simulink model "reconfig_dev_2021a"  (R2021a)
settings: Solver=VariableStepAuto  StartTime=0.0  StopTime=tsim  RelTol=1e-3
InitFcn:
  | main
values from neighbouring files (symbols this model uses):
  drone_params = get_parameters(1)    [main.m]
  dt = 0.005    [main.m]
  g = 9.81    [main.m]
  gust_duration = 5    [main.m]
  gust_force = [0;0;0]    [main.m]
  gust_start = 8    [main.m]
  omega0 = [[0,0,0]',[0,0,0]',[0,0,0]']    [main.m]
  p0 = [[0,0,2]',[0,0,2]',[0,0,2]']    [main.m]
  q0 = [[1,0,0,0]',[1,0,0,0]',[1,0,0,0]']    [main.m]
  tsim = 10    [main.m]
  v0 = [[0,0,0]',[0,0,0]',[0,0,0]']    [main.m]
libraries: vrlib x1
settings Model: Creator=gbattaglia2021  LastModifiedBy=Giacomo Battaglia

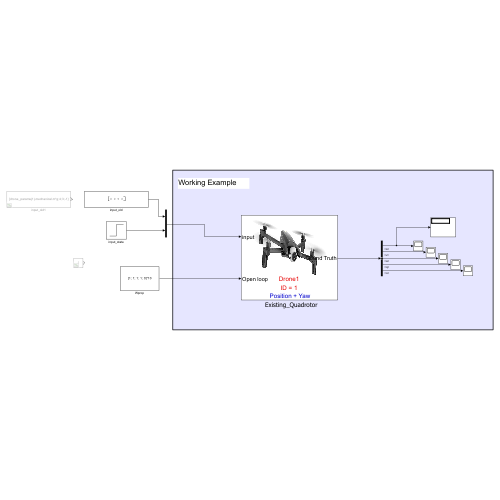
[thumbnail: Simulink's stored preview of the top-level diagram]
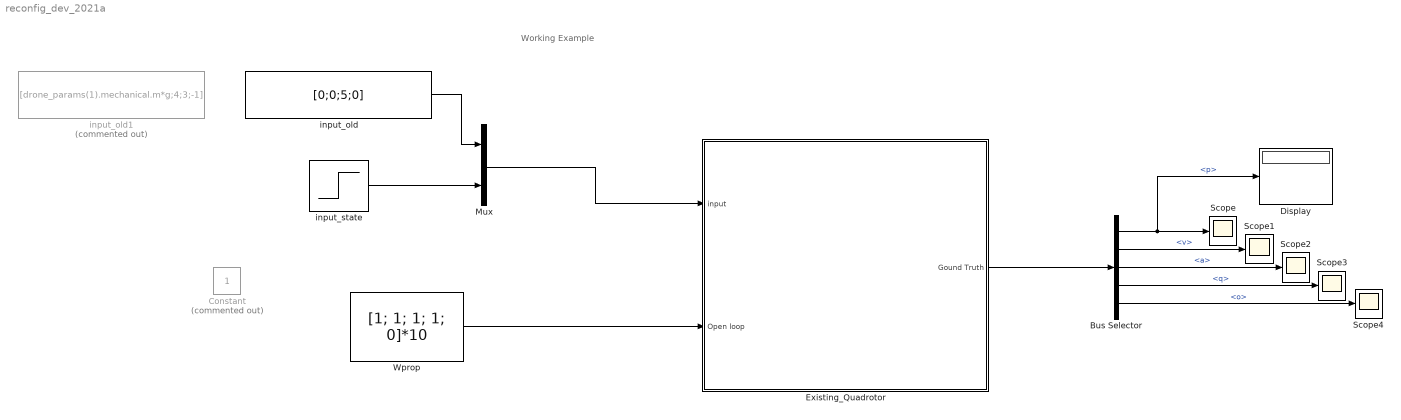
== system reconfig_dev_2021a ==
  note: Working Example
  "  Existing_Quadrotor" : Subsystem  mask{control_type_param=1: Position + Yaw, DroneID=1, DroneName=Drone1, idx_offset=0}
      mask prompts: control_type_param "Controller type"; DroneName "Drone Name"; idx_offset "Index Offset"
      mask TypeOptions control_type_param: 1: Position + Yaw | 2: Body Velocity + Yawrate | 3: Body Acceleration + Yawrate | 4: Thrust + Attitude | 5: Thrust + Body Rate | 6: Body Wrench
      mask TypeOptions DroneID: 1 | 2 | 3 | 4 | 5 | 6 | 7 | 8 | 9
      mask Callback DroneID:
      | ID = get_param(gcb,'DroneID');
      | offset = get_param(gcb,'idx_offset');
      | if ischar(ID)
      |   ID = str2num(ID);
      | end
      | if ischar(offset)
      |   offset = str2num(offset);
      | end
      | nameID = ID + offset;
      | set_param(gcb,'DroneName',["Drone"+num2str(nameID)]);
      mask Callback DroneName: set_param([gcb,'/To Workspace'],'VariableName',[get_param(gcb,'DroneName')]);
      mask Callback idx_offset:
      | ID = get_param(gcb,'DroneID');
      | offset = get_param(gcb,'idx_offset');
      | if ischar(ID)
      |   ID = str2num(ID);
      | end
      | if ischar(offset)
      |   offset = str2num(offset);
      | end
      | nameID = ID + offset;
      | set_param(gcb,'DroneName',["Drone"+num2str(nameID)]);
      mask DialogControl Control4 Prompt: click to choose controller
      mask Display:
      | image('format/drone_image.png'); % Use "Edit Image" on toolstrip to change.
      | Name = get_param(gcb,'DroneName');
      | ID = get_param(gcb,'DroneID');
      | C_mode = get_param(gcb,'control_type_param');
      | C_mode(1:2) = [];
      | color('red')
      | ID = "ID = "+ID;
      | color('red')
      | text(0.5, 0.25, Name, 'horizontalAlignment', 'center')
      | color('red')
      | text(0.5, 0.15, ID, 'horizontalAlignment', 'center')
      | color('blue');
      | text(0.5, 0.05, C_mode, 'horizontalAlignment', 'center')
  Bus Selector : BusSelector  OutputSignals=p,v,a,q,o
  Constant : Constant  Commented=on
  Display : Display
  Mux : Mux  Inputs=2
  Scope{,1..4} (5 alike) : Scope
  Wprop : Constant  Value=[1; 1; 1; 1; 0]*10
  input_old : Constant  Value=[0;0;5;0]
  input_old1 : Constant  Commented=on  Value=[drone_params(1).mechanical.m*g;4;3;-1]
  input_state : Step  Time=tsim/2  Before=drone_params(1).control.state  After=drone_params(1).control.state_enum.folded2  SampleTime=0
  wires:
  Bus Selector/1 -> Display/1, Scope/1  "<p>"
  Bus Selector/4 -> Scope3/1  "<q>"
  Bus Selector/5 -> Scope4/1  "<o>"
  Bus Selector/2 -> Scope1/1  "<v>"
  "  Existing_Quadrotor"/1(Gound Truth) -> Bus Selector/1
  Bus Selector/3 -> Scope2/1  "<a>"
  Wprop/1 -> "  Existing_Quadrotor"/2(Open loop)
  input_old/1 -> Mux/1
  Mux/1 -> "  Existing_Quadrotor"/1(input)
  input_state/1 -> Mux/2

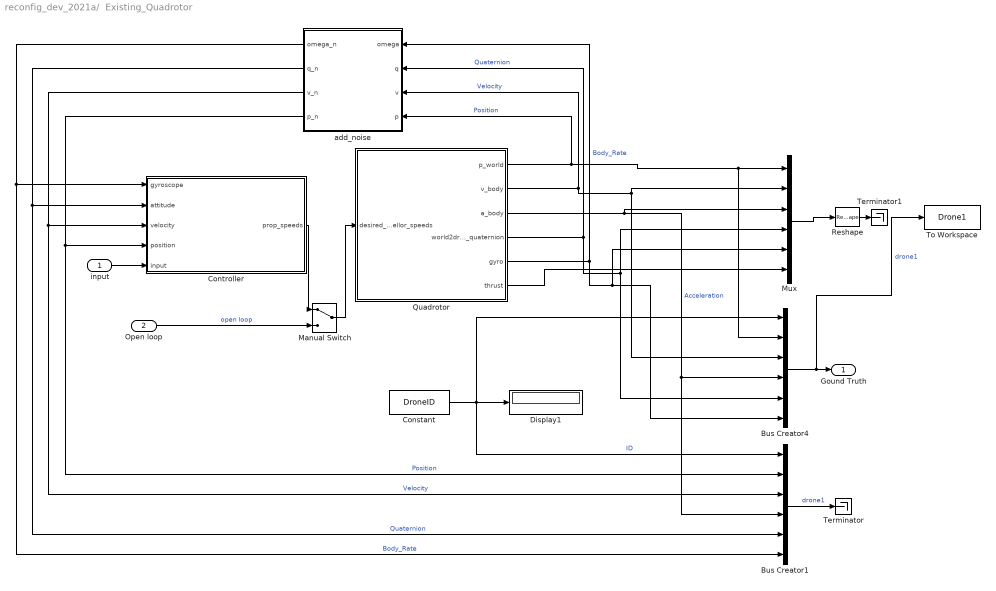
== system reconfig_dev_2021a/  Existing_Quadrotor ==
  input : Inport
  Open loop : Inport  Port=2
  Bus Creator1 : BusCreator  Inputs=6  OutDataTypeStr=Bus: DroneStateBus
      settings: InheritFromInputs=off
  Bus Creator4 : BusCreator  Inputs=6  OutDataTypeStr=Bus: DroneStateBus
      settings: InheritFromInputs=off
  Constant : Constant  Value=DroneID
  Controller : Subsystem
  Display1 : Display
  Manual Switch : ManualSwitch
  Mux : Mux  Inputs=6
  Quadrotor : Subsystem
      mask Display: image('droneHardware.jpeg'); % Use "Edit Image" on toolstrip to change.
  Reshape : Reshape
  Terminator : Terminator
  Terminator1 : Terminator
  To Workspace : ToWorkspace  VariableName=Drone1  SaveFormat=Timeseries  SampleTime=-1
  add_noise : MATLAB Function  TreatAsAtomicUnit=on
  Gound Truth : Outport
  wires:
  Quadrotor/5(gyro) -> add_noise/1(omega), Bus Creator4/6, Mux/5  "Body_Rate"
  Quadrotor/1(p_world) -> add_noise/4(p), Bus Creator4/2, Mux/1  "Position"
  Quadrotor/4(world2drone_quaternion) -> add_noise/2(q), Bus Creator4/5, Mux/4  "Quaternion"
  Mux/1 -> Reshape/1
  Quadrotor/2(v_body) -> add_noise/3(v), Bus Creator4/3, Mux/2  "Velocity"
  Quadrotor/6(thrust) -> Mux/6
  input/1 -> Controller/5(input)
  Bus Creator4/1 -> To Workspace/1, Gound Truth/1  "drone1"
  add_noise/2(q_n) -> Bus Creator1/5, Controller/2(attitude)  "Quaternion"
  Quadrotor/3(a_body) -> Mux/3, Bus Creator4/4, Bus Creator1/4  "Acceleration"
  Bus Creator1/1 -> Terminator/1  "drone1"
  add_noise/4(p_n) -> Bus Creator1/2, Controller/4(position)  "Position"
  add_noise/3(v_n) -> Controller/3(velocity), Bus Creator1/3  "Velocity"
  Constant/1 -> Bus Creator4/1, Display1/1, Bus Creator1/1  "ID"
  add_noise/1(omega_n) -> Controller/1(gyroscope), Bus Creator1/6  "Body_Rate"
  Reshape/1 -> Terminator1/1
  Manual Switch/1 -> Quadrotor/1(desired_propellor_speeds)
  Controller/1(prop_speeds) -> Manual Switch/1
  Open loop/1 -> Manual Switch/2  "open loop"

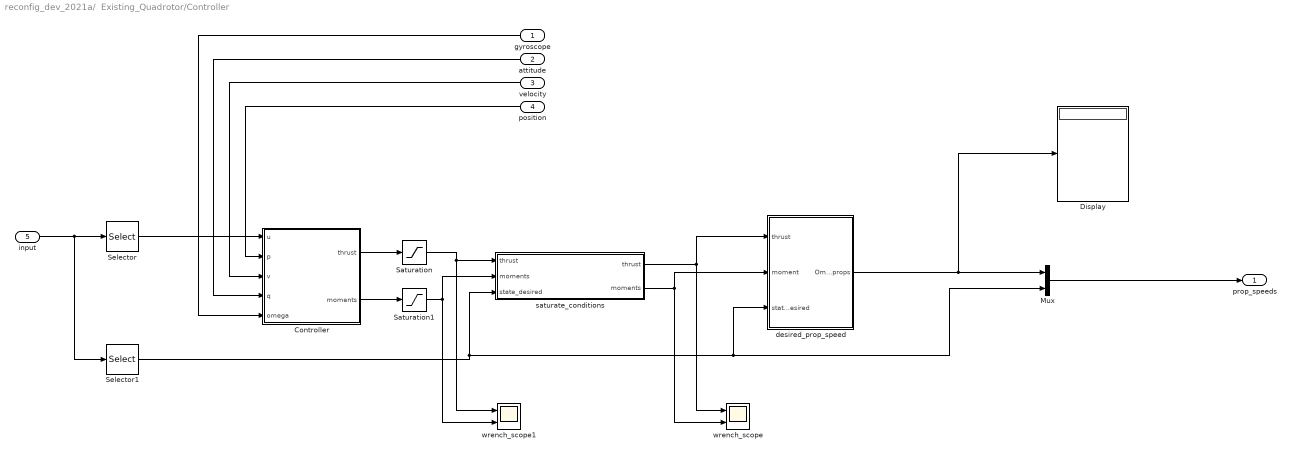
== system reconfig_dev_2021a/  Existing_Quadrotor/Controller ==
  gyroscope : Inport
  attitude : Inport  Port=2
  velocity : Inport  Port=3
  position : Inport  Port=4
  input : Inport  Port=5
  Controller : MATLAB Function  TreatAsAtomicUnit=on
  Display : Display
  Mux : Mux  Inputs=2
  Saturation : Saturate  UpperLimit=16  LowerLimit=3
  Saturation1 : Saturate  UpperLimit=0.1  LowerLimit=-0.1
  Selector : Selector  InputPortWidth=5  IndexOptions=Index vector (dialog)  Indices=[1 2 3 4]  OutputSizes=1
  Selector1 : Selector  InputPortWidth=5  IndexOptions=Index vector (dialog)  Indices=[5]  OutputSizes=1
  desired_prop_speed : MATLAB Function  TreatAsAtomicUnit=on
  saturate_conditions : MATLAB Function  TreatAsAtomicUnit=on
  wrench_scope : Scope  NumInputPorts=2
  wrench_scope1 : Scope  NumInputPorts=2
  prop_speeds : Outport
  wires:
  Controller/2(moments) -> Saturation1/1
  velocity/1 -> Controller/3(v)
  Controller/1(thrust) -> Saturation/1
  position/1 -> Controller/2(p)
  attitude/1 -> Controller/4(q)
  gyroscope/1 -> Controller/5(omega)
  desired_prop_speed/1(Omega_props) -> Mux/1, Display/1
  Saturation/1 -> wrench_scope1/1, saturate_conditions/1("thrust ")
  Saturation1/1 -> wrench_scope1/2, saturate_conditions/2("moments ")
  saturate_conditions/1(thrust) -> wrench_scope/1, desired_prop_speed/1(thrust)
  saturate_conditions/2(moments) -> wrench_scope/2, desired_prop_speed/2(moment)
  Selector1/1 -> Mux/2, desired_prop_speed/3(state_desired), saturate_conditions/3(state_desired)
  input/1 -> Selector1/1, Selector/1
  Selector/1 -> Controller/1(u)
  Mux/1 -> prop_speeds/1

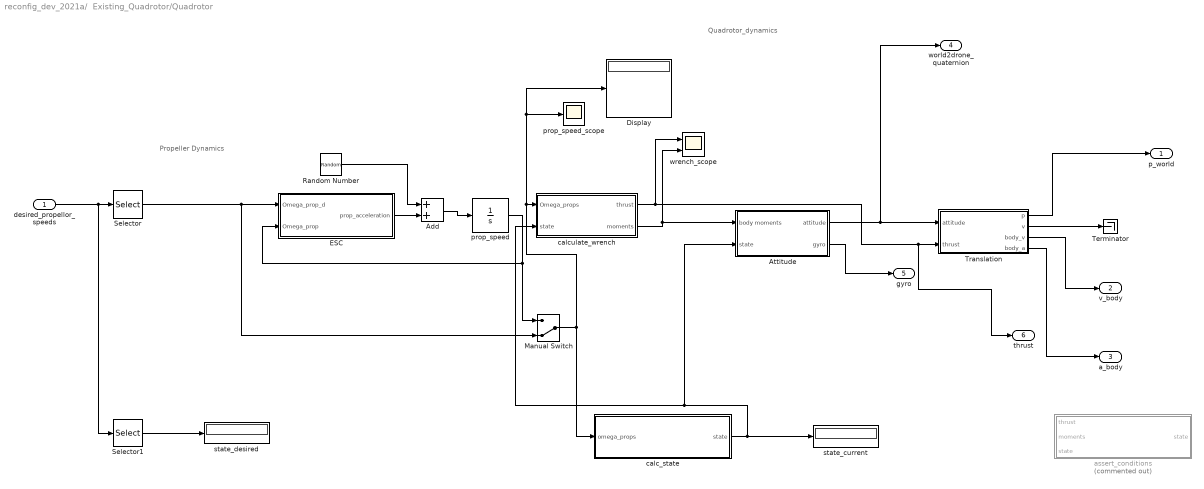
== system reconfig_dev_2021a/  Existing_Quadrotor/Quadrotor ==
  note: Quadrotor_dynamics
  note: Propeller Dynamics
  desired_propellor_speeds : Inport
  Add : Sum
  Attitude : Subsystem
  Display : Display
  ESC : MATLAB Function  TreatAsAtomicUnit=on
  Manual Switch : ManualSwitch  CurrentSetting=0
  Random Number : RandomNumber  Mean=[0;0;0;0]  Variance=[5000;5000;5000;5000]  Seed=[1;2;3;4]  SampleTime=dt
  Selector : Selector  InputPortWidth=5  IndexOptions=Index vector (dialog)  Indices=[1 2 3 4]  OutputSizes=1
  Selector1 : Selector  InputPortWidth=5  IndexOptions=Index vector (dialog)  Indices=[5]  OutputSizes=1
  Terminator : Terminator
  Translation : Subsystem
  assert_conditions : MATLAB Function  Commented=on  TreatAsAtomicUnit=on
  calc_state : MATLAB Function  TreatAsAtomicUnit=on
  calculate_wrench : MATLAB Function  TreatAsAtomicUnit=on
  prop_speed : Integrator  InitialCondition=drone_params(DroneID).motors.omega0  LimitOutput=on  UpperSaturationLimit=drone_params(DroneID).motors.omega_max  LowerSaturationLimit=drone_params(DroneID).motors.omega_min
  prop_speed_scope : Scope
  state_current : Display
  state_desired : Display
  wrench_scope : Scope  NumInputPorts=2
  p_world : Outport
  v_body : Outport  Port=2
  a_body : Outport  Port=3
  world2drone_quaternion : Outport  Port=4
  gyro : Outport  Port=5
  thrust : Outport  Port=6
  wires:
  calculate_wrench/1(thrust) -> wrench_scope/1, thrust/1, Translation/2(thrust)
  Add/1 -> prop_speed/1
  desired_propellor_speeds/1 -> Selector1/1, Selector/1
  prop_speed/1 -> Manual Switch/1, ESC/2(Omega_prop)
  calculate_wrench/2(moments) -> wrench_scope/2, Attitude/1(body moments)
  Attitude/1(attitude) -> world2drone_quaternion/1, Translation/1(attitude)
  Attitude/2(gyro) -> gyro/1
  Translation/3(body_v) -> v_body/1
  Translation/4(body_a) -> a_body/1
  Translation/1(p) -> p_world/1
  Random Number/1 -> Add/1
  ESC/1(prop_acceleration) -> Add/2
  Manual Switch/1 -> Display/1, prop_speed_scope/1, calculate_wrench/1(Omega_props), calc_state/1(omega_props)
  Translation/2(v) -> Terminator/1
  Selector/1 -> Manual Switch/2, ESC/1(Omega_prop_d)
  Selector1/1 -> state_desired/1
  calc_state/1(state) -> state_current/1, Attitude/2(state), calculate_wrench/2(state)

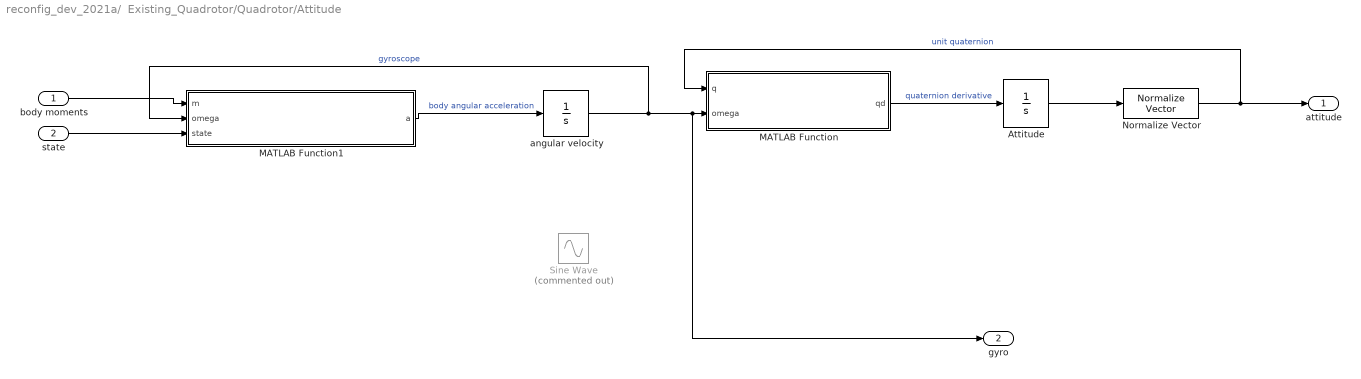
== system reconfig_dev_2021a/  Existing_Quadrotor/Quadrotor/Attitude ==
  body moments : Inport
  state : Inport  Port=2
  Attitude : Integrator  InitialCondition=q0(:,DroneID)
  MATLAB Function : MATLAB Function  TreatAsAtomicUnit=on
  MATLAB Function1 : MATLAB Function  TreatAsAtomicUnit=on
  Normalize Vector : vrlib/Utilities/Normalize Vector  maxzero=0
  Sine Wave : Sin  Commented=on  Amplitude=[0.5;0.5;0.5]  Frequency=[1;0.3;0.6]  SampleTime=0
  angular velocity : Integrator  InitialCondition=omega0(:,DroneID)
  attitude : Outport
  gyro : Outport  Port=2
  wires:
  Attitude/1 -> Normalize Vector/1
  MATLAB Function/1(qd) -> Attitude/1  "quaternion derivative"
  body moments/1 -> MATLAB Function1/1(m)
  MATLAB Function1/1(a) -> angular velocity/1  "body angular acceleration"
  angular velocity/1 -> gyro/1, MATLAB Function/2(omega), MATLAB Function1/2(omega)  "gyroscope"
  Normalize Vector/1 -> MATLAB Function/1(q), attitude/1  "unit quaternion"
  state/1 -> MATLAB Function1/3(state)

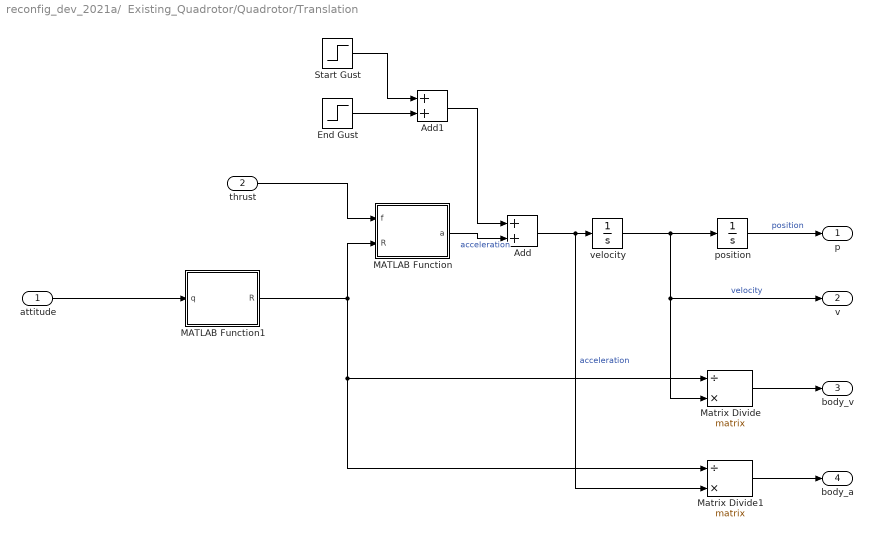
== system reconfig_dev_2021a/  Existing_Quadrotor/Quadrotor/Translation ==
  attitude : Inport
  thrust : Inport  Port=2
  Add : Sum
  Add1 : Sum
  End Gust : Step  Time=gust_start + gust_duration  Before=[0;0;0]  After=-1*gust_force/drone_params(DroneID).mechanical.m  SampleTime=0
  MATLAB Function : MATLAB Function  TreatAsAtomicUnit=on
  MATLAB Function1 : MATLAB Function  TreatAsAtomicUnit=on
  Matrix Divide : Product  Inputs=/*  Multiplication=Matrix(*)
  Matrix Divide1 : Product  Inputs=/*  Multiplication=Matrix(*)
  Start Gust : Step  Time=gust_start  Before=[0;0;0]  After=gust_force/drone_params(DroneID).mechanical.m  SampleTime=0
  position : Integrator  InitialCondition=p0(:,DroneID)
  velocity : Integrator  InitialCondition=v0(:,DroneID)
  p : Outport
  v : Outport  Port=2
  body_v : Outport  Port=3
  body_a : Outport  Port=4
  wires:
  velocity/1 -> Matrix Divide/2, v/1, position/1  "velocity"
  position/1 -> p/1  "position"
  Add/1 -> Matrix Divide1/2, velocity/1  "acceleration"
  attitude/1 -> MATLAB Function1/1(q)
  thrust/1 -> MATLAB Function/1(f)
  MATLAB Function1/1(R) -> Matrix Divide1/1, Matrix Divide/1, MATLAB Function/2(R)
  Matrix Divide/1 -> body_v/1
  Matrix Divide1/1 -> body_a/1
  MATLAB Function/1(a) -> Add/2  "acceleration"
  Add1/1 -> Add/1
  End Gust/1 -> Add1/2
  Start Gust/1 -> Add1/1

== matlab function reconfig_dev_2021a/  Existing_Quadrotor/Quadrotor/ESC ==
  data: Omega_prop_d input; prop_acceleration output; Omega_prop input; DroneID parameter; drone_params parameter
function prop_acceleration  =  ESC_ctrl(Omega_prop_d, Omega_prop, DroneID, drone_params)

prop_acceleration = (Omega_prop_d - Omega_prop)*drone_params(DroneID).motors.gain;

== matlab function reconfig_dev_2021a/  Existing_Quadrotor/Quadrotor/Translation/MATLAB Function ==
  data: f input; a output; R input; g parameter; drone_params parameter; DroneID parameter
function a = fcn(f, R, g, drone_params, DroneID)
m = drone_params(DroneID).mechanical.m;
a = R*[0;0;f]/m - [0;0;g];

== matlab function reconfig_dev_2021a/  Existing_Quadrotor/Quadrotor/Translation/MATLAB Function1 ==
  data: q input; R output
function R = quat2rotm(q)
  R = eye(3);
  coder.extrinsic('quat2rotm.m');
  R = quat2rotm(q);
end

== matlab function reconfig_dev_2021a/  Existing_Quadrotor/Quadrotor/calculate_wrench ==
  data: Omega_props input; state input; thrust output; moments output; drone_params parameter; DroneID parameter
function [thrust, moments] =  invAllocation(Omega_props, state, drone_params, DroneID)

M = drone_params(DroneID).control.allocation_matrix;
if state ~= drone_params(DroneID).control.state
switch state
    case drone_params(DroneID).control.state_enum.unfolded
        M = drone_params(DroneID).control.allocation_matrix_u;
    case drone_params(DroneID).control.state_enum.folded2
        M = drone_params(DroneID).control.allocation_matrix_2f;
    case drone_params(DroneID).control.state_enum.folded4
        M = drone_params(DroneID).control.allocation_matrix_4f;
end
end

wrench = M*(Omega_props.^2);

thrust = wrench(1);
moments = wrench(2:4);

== matlab function reconfig_dev_2021a/  Existing_Quadrotor/add_noise ==
  settings: updateMethod=DISCRETE
  data: omega input; omega_n output size=3; q input; v input; p input; q_n output size=4; v_n output size=3; p_n output size=3; drone_params parameter; DroneID parameter
function [omega_n, q_n, v_n, p_n]= add_noise(omega,q,v,p, drone_params, DroneID)

omega_n = omega + drone_params(DroneID).sensor.gyroscope_noise*(rand(3,1)-0.5);

q_n = q + drone_params(DroneID).sensor.attitude_noise*(rand(4,1)-0.5);
q_n = q_n/norm(q_n);

v_n = v + drone_params(DroneID).sensor.velocity_noise*(rand(3,1)-0.5);

p_n = p + drone_params(DroneID).sensor.position_noise*(rand(3,1)-0.5);

end

== matlab function reconfig_dev_2021a/  Existing_Quadrotor/Controller/saturate_conditions ==
  data: thrust input; moments input; state_desired input; drone_params parameter; DroneID parameter; thrust output; moments output
function [thrust, moments] = saturate_conditions(thrust, moments, state_desired, drone_params, DroneID)

coder.extrinsic("solve_conditions");
coder.extrinsic("verify_conditions");
[verify_u, verify_2f] = verify_conditions(thrust,moments);

if state_desired == drone_params(DroneID).control.state_enum.unfolded
    if (verify_u)
        return;
    end
    moments(3) = solve_conditions(thrust,moments,"u");

elseif state_desired == drone_params(DroneID).control.state_enum.folded2
   if (~verify_u && verify_2f)
        return;
   end
   moments(3) = solve_conditions(thrust,moments,"2f");

elseif state_desired == drone_params(DroneID).control.state_enum.folded4
   if (~verify_u && ~verify_2f)
        return;
   end


end

== matlab function reconfig_dev_2021a/  Existing_Quadrotor/Quadrotor/calc_state ==
  data: omega_props input; drone_params parameter; DroneID parameter; state output
function state = calculate_state(omega_props, drone_params, DroneID)

omega_indicator = omega_props >= 0;

if sum(omega_indicator) == 4
%     disp("Passing to u");
    state = drone_params(DroneID).control.state_enum.unfolded;
elseif sum(omega_indicator) == 2
%     disp("Passing to 2f");
    state = drone_params(DroneID).control.state_enum.folded2;
else
%     disp("Passing to 4f");
    state = drone_params(DroneID).control.state_enum.folded4;
% else
%     disp("WARNING: not possible condition");
%     state = drone_params(DroneID).control.state_enum.unfolded;
end

== matlab function reconfig_dev_2021a/  Existing_Quadrotor/Quadrotor/assert_conditions ==
  data: thrust input; moments input; state input; drone_params parameter; DroneID parameter; state output
function state = assert_conditions(thrust, moments, state, drone_params, DroneID)

coder.extrinsic("verify_conditions");
[verify_u,verify_2f] = verify_conditions(thrust,moments);

if state == drone_params(DroneID).control.state_enum.unfolded
    if verify_u
       return;
    elseif verify_2f
        disp("Passing to 2f");
        drone_params(DroneID).mechanical.I = drone_params(DroneID).mechanical.I2f;
        state = drone_params(DroneID).control.state_enum.folded2;
%         drone_params(DroneID).control.allocation_matrix = drone_params(DroneID).control.allocation_matrix_2f;
    else
        disp("Passing to 4f");
        drone_params(DroneID).mechanical.I = drone_params(DroneID).mechanical.I4f;
        state = drone_params(DroneID).control.state_enum.folded4;
%         drone_params(DroneID).control.allocation_matrix = drone_params(DroneID).control.allocation_matrix_4f;
    end
elseif state == drone_params(DroneID).control.state_enum.folded2
    if verify_u
       disp("Passing to u");
       drone_params(DroneID).mechanical.I = drone_params(DroneID).mechanical.Iu;
       state = drone_params(DroneID).control.state_enum.unfolded;
%        drone_params(DroneID).control.allocation_matrix = drone_params(DroneID).control.allocation_matrix_u;
    elseif verify_2f
        return;
    else
        disp("Passing to 4f");
        drone_params(DroneID).mechanical.I = drone_params(DroneID).mechanical.I4f;
        state = drone_params(DroneID).control.state_enum.folded4;
%         drone_params(DroneID).control.allocation_matrix = drone_params(DroneID).control.allocation_matrix_4f;
    end
elseif state == drone_params(DroneID).control.state_enum.folded4
    if verify_u
        disp("Passing to u");
        drone_params(DroneID).mechanical.I = drone_params(DroneID).mechanical.Iu;
        drone_params(DroneID).control.state = drone_params(DroneID).control.state_enum.unfolded;
%         drone_params(DroneID).control.allocation_matrix = drone_params(DroneID).control.allocation_matrix_u;
    elseif verify_2f
        disp("Passing to 2f");
        drone_params(DroneID).mechanical.I = drone_params(DroneID).mechanical.I2f;
        state = drone_params(DroneID).control.state_enum.folded2;
%         drone_params(DroneID).control.allocation_matrix = drone_params(DroneID).control.allocation_matrix_2f;
    else
       return; 
    end
end

== matlab function reconfig_dev_2021a/  Existing_Quadrotor/Controller/Controller ==
  data: u input; p input size=3; v input size=3; q input size=4; omega input size=3; thrust output size=1; moments output size=3; control_type_param parameter; drone_params parameter; DroneID parameter; g parameter
function [thrust, moments] = controller(u, p, v, q, omega, control_type_param, drone_params, DroneID, g)

    thrust = 1; % set output dim
    moments = [0;0;0]; % set output dim

  coder.extrinsic('droneControl'); % link simulink to matlab function
  
  % do control
  [thrust, moments] = droneControl(u, p, v, q, omega, ...
    control_type_param, drone_params, DroneID, g);


end

== matlab function reconfig_dev_2021a/  Existing_Quadrotor/Controller/desired_prop_speed ==
  data: thrust input; Omega_props output; moment input; state_desired input; drone_params parameter; DroneID parameter
function Omega_props  =  Allocation(thrust, moment, state_desired, drone_params, DroneID)

M = drone_params(DroneID).control.allocation_matrix;
if state_desired ~= drone_params(DroneID).control.state
switch state_desired
    case drone_params(DroneID).control.state_enum.unfolded
        M = drone_params(DroneID).control.allocation_matrix_u;
    case drone_params(DroneID).control.state_enum.folded2
        M = drone_params(DroneID).control.allocation_matrix_2f;
    case drone_params(DroneID).control.state_enum.folded4
        M = drone_params(DroneID).control.allocation_matrix_4f;
end
end

%  Omega_props = sqrt(inv(alloc_mat) * [thrust;moment]);
if state_desired ~= drone_params(DroneID).control.state_enum.folded4
    W2 = M \ [thrust;moment];
    Omega_props = real(sqrt(complex(W2)));
else
    W2 = pinv(M(2:4,:)) * moment;
    Omega_props = real(sqrt(complex(W2)));
end

if state_desired == drone_params(DroneID).control.state_enum.folded2
    Omega_props = Omega_props.*[-1; -1; 1; 1];
elseif state_desired == drone_params(DroneID).control.state_enum.folded4
    Omega_props = Omega_props.*[-1; -1; -1; -1];
end

== matlab function reconfig_dev_2021a/  Existing_Quadrotor/Quadrotor/Attitude/MATLAB Function ==
  data: q input size=4; omega input size=3; qd output size=4
function qd  = quaternion_derivative(q, omega)


qd =  0.5 * multiplyQuaternions([0;omega],q);

end


function q = multiplyQuaternions(qA,qB)
q0 = qA(1);
q1 = qA(2);
q2 = qA(3);
q3 = qA(4);
Q = [q0, -q1, -q2, -q3;
     q1,  q0, -q3,  q2;
     q2,  q3,  q0, -q1;
     q3, -q2,  q1,  q0];
q = Q * qB;
end

== matlab function reconfig_dev_2021a/  Existing_Quadrotor/Quadrotor/Attitude/MATLAB Function1 ==
  data: m input; a output; omega input; state input; drone_params parameter; DroneID parameter
function a = moments2angularacceleration(m, omega, state, drone_params, DroneID)

I = drone_params(DroneID).mechanical.I;
switch state
    case drone_params(DroneID).control.state_enum.unfolded
        I = drone_params(DroneID).mechanical.Iu;
    case drone_params(DroneID).control.state_enum.folded2
        I = drone_params(DroneID).mechanical.I2f;
    case drone_params(DroneID).control.state_enum.folded4
        I = drone_params(DroneID).mechanical.I4f;
end

a = inv(I)*m  - inv(I) * cross(omega,I*omega);
